simulink model "blade_liebherr_2021_05_26"  (R2020a)
settings: Solver=ode23tb  StartTime=0.0  StopTime=simulation_length  MaxStep=tsample
values from neighbouring files (symbols this model uses):
  tsample = 1e-3    (= 0.001)    [init_liebherr_blade.m]
libraries: nesl_utility x52, fl_lib x31, bichamber_piston_lib x5, fourway_threeland_valve_lib x3, fourway_fourland_valve_lib x2, engine_speed_ctrl_lib x1, Liebherr_Engine_D934_lib x1, pressure_controlled_pump_lib x1
settings Model: SimulationMode=accelerator  Creator=dbagn  LastModifiedBy=dbagn
settings SolverCC: ZeroCrossControl=DisableAll  ZeroCrossAlgorithm=Adaptive
settings DataIOCC: SaveTime=off  ReturnWorkspaceOutputs=off
settings DebuggingCC: IgnoredZcDiagnostic=none
settings SFSimCC: SimParseCustomCode=off

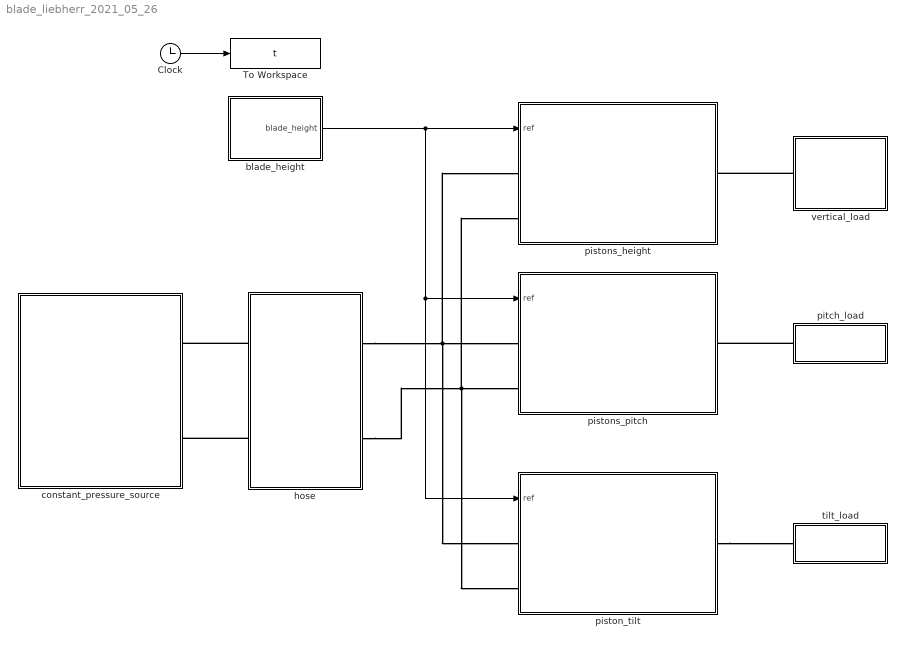
== system blade_liebherr_2021_05_26 ==
  Clock : Clock
  To Workspace : ToWorkspace  VariableName=t  SampleTime=tsample
      settings: MaxDataPoints=Nsample
  blade_height : Subsystem
  constant_pressure_source : Subsystem
  hose : Subsystem
  piston_tilt : Subsystem
  pistons_height : Subsystem
  pistons_pitch : Subsystem
  pitch_load : Subsystem
  tilt_load : Subsystem
  vertical_load : Subsystem
  wires:
  Clock/1 -> To Workspace/1
  blade_height/1(blade_height) -> piston_tilt/1(ref), pistons_pitch/1(ref), pistons_height/1(ref)
  connections:
  hose/LConn1 -- constant_pressure_source/RConn1
  hose/LConn2 -- constant_pressure_source/RConn2
  hose/RConn1 -- piston_tilt/LConn1 -- pistons_height/LConn1 -- pistons_pitch/LConn1
  hose/RConn2 -- piston_tilt/LConn2 -- pistons_height/LConn2 -- pistons_pitch/LConn2
  vertical_load/LConn1 -- pistons_height/RConn1
  pitch_load/RConn1 -- pistons_pitch/RConn1
  piston_tilt/RConn1 -- tilt_load/RConn1

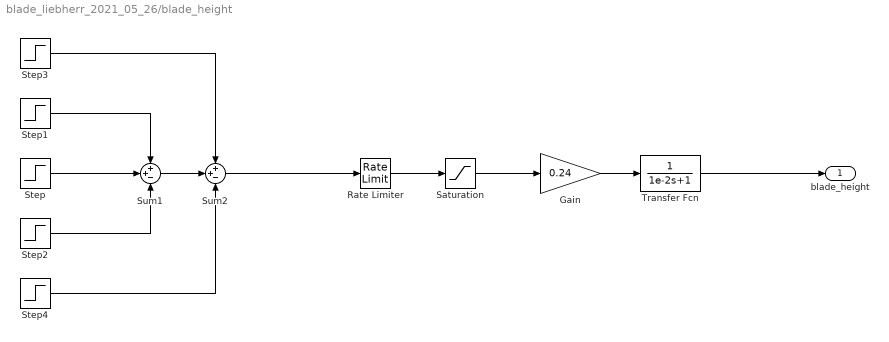
== system blade_liebherr_2021_05_26/blade_height ==
  Gain : Gain  Gain=0.24
  Rate Limiter : RateLimiter  RisingSlewLimit=0.2  FallingSlewLimit=-0.2  SampleTimeMode=inherited
  Saturation : Saturate  UpperLimit=0.99  LowerLimit=-0.99
  Step : Step  Time=20  After=0.5  SampleTime=0
  Step1 : Step  Time=40  SampleTime=0
  Step2 : Step  Time=60  After=2.5  SampleTime=0
  Step3 : Step  Time=80  After=1.4  SampleTime=0
  Step4 : Step  Time=100  After=-0.5  SampleTime=0
  Sum1 : Sum  Inputs=++-
  Sum2 : Sum  Inputs=++-
  Transfer Fcn : TransferFcn  Denominator=[1e-2 1]
  blade_height : Outport
  wires:
  Step/1 -> Sum1/2
  Gain/1 -> Transfer Fcn/1
  Transfer Fcn/1 -> blade_height/1
  Step1/1 -> Sum1/1
  Step2/1 -> Sum1/3
  Sum1/1 -> Sum2/2
  Step3/1 -> Sum2/1
  Step4/1 -> Sum2/3
  Saturation/1 -> Gain/1
  Sum2/1 -> Rate Limiter/1
  Rate Limiter/1 -> Saturation/1

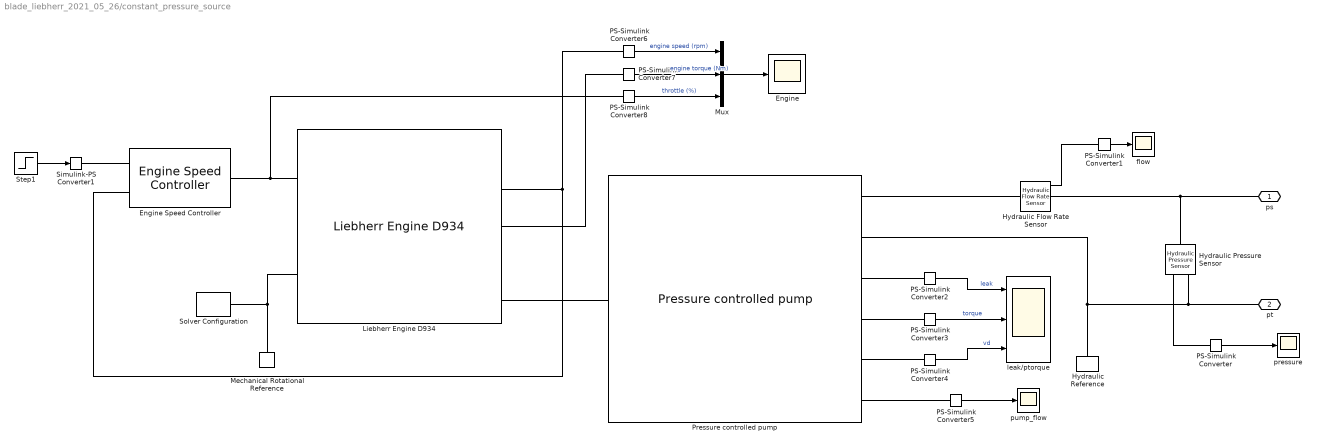
== system blade_liebherr_2021_05_26/constant_pressure_source ==
  Engine : Scope
  Engine Speed Controller : engine_speed_ctrl_lib/Engine Speed Controller  kp=1e-1 s  kint=1e-2  kd=0 s^2  t_out_specify=off  t_out_priority=High  t_out=0  t_out_nominal_specify=off  t_out_nominal_unit=1  t_out_nominal_value=1
      settings: InternalSimscapePortConfiguration="{\"Bottom\":[],\"Left\":[{\"id\":\"we_ref\",\"label\":\"we_ref\",\"type\":\"input\"},{\"id\":\"we\",\"label\":\"we\",\"type\":\"input\"}],\"Right\":[{\"id\":\"theta\",\"label\":\"theta\",\"type\":\"output\"}],\"Top\":[]}"
  Hydraulic Flow Rate Sensor : fl_lib/Hydraulic/Hydraulic Sensors/Hydraulic Flow Rate Sensor
  Hydraulic Pressure Sensor : fl_lib/Hydraulic/Hydraulic Sensors/Hydraulic Pressure Sensor
  Hydraulic Reference : fl_lib/Hydraulic/Hydraulic Elements/Hydraulic Reference
  Liebherr Engine D934 : Liebherr_Engine_D934_lib/Liebherr Engine D934  dynamic_response=simscape.enum.onoff.on  cshaft_inertia=7.5 kg*m^2  initial_speed=600
      settings: InternalSimscapePortConfiguration="{\"Bottom\":[],\"Left\":[{\"id\":\"tS\",\"label\":\"tS\",\"type\":\"input\"},{\"id\":\"C\",\"label\":\"C\",\"type\":\"foundation.mechanical.rotational.rotational\"}],\"Right\":[{\"id\":\"PE\",\"label\":\"PE\",\"type\":\"output\"},{\"id\":\"wE\",\"label\":\"wE\",\"type\":\"output\"},{\"id\":\"tE\",\"label\":\"tE\",\"type\":\"output\"},{\"id\":\"eE\",\"label\":\"eE\",\"type\":\"output\"},{\"id\":\"D\",\"label\":\"D\",\"type\":\"foundation.mechanical.rotational.rotational\"}],\"Top\":[]}"
  Mechanical Rotational Reference : fl_lib/Mechanical/Rotational Elements/Mechanical Rotational Reference
  Mux : Mux  Inputs=3
  PS-Simulink Converter : nesl_utility/PS-Simulink Converter  PhysicalDomain=network_engine_domain  SubClassName=ps_output  LeftPortType=input  RightPortType=output  PseudoPeriodic=off  Frequencies=[]  Unit=bar  AffineConversion=on
  PS-Simulink Converter1 : nesl_utility/PS-Simulink Converter  PhysicalDomain=network_engine_domain  SubClassName=ps_output  LeftPortType=input  RightPortType=output  PseudoPeriodic=off  Frequencies=[]  Unit=l/min  AffineConversion=on
  PS-Simulink Converter{2..5} (4 alike) : nesl_utility/PS-Simulink Converter  PhysicalDomain=network_engine_domain  SubClassName=ps_output  LeftPortType=input  RightPortType=output  PseudoPeriodic=off  Frequencies=[]  Unit=1  AffineConversion=off
  PS-Simulink Converter6 : nesl_utility/PS-Simulink Converter  PhysicalDomain=network_engine_domain  SubClassName=ps_output  LeftPortType=input  RightPortType=output  PseudoPeriodic=off  Frequencies=[]  Unit=inherit  AffineConversion=off
  PS-Simulink Converter7 : nesl_utility/PS-Simulink Converter  PhysicalDomain=network_engine_domain  SubClassName=ps_output  LeftPortType=input  RightPortType=output  PseudoPeriodic=off  Frequencies=[]  Unit=inherit  AffineConversion=off
  PS-Simulink Converter8 : nesl_utility/PS-Simulink Converter  PhysicalDomain=network_engine_domain  SubClassName=ps_output  LeftPortType=input  RightPortType=output  PseudoPeriodic=off  Frequencies=[]  Unit=inherit  AffineConversion=off
  Pressure controlled pump : pressure_controlled_pump_lib/Pressure controlled pump  Vd_nom=62.3*10 cm^3/rev  dp_ref=250 bar  pnom=250 bar  b=0.1 N*m/(rad/s)  inertia_pump=0.027 kg*m^2  vd_lim_max=0.98  vd_lim_min=0  p_set=258 bar  p_reg=8 bar  x_rv_max=12 mm  kpc=8  kic=8 1/s  te_specify=off  te_priority=None  te=0 N*m  te_nominal_specify=off  te_nominal_unit=N*m  te_nominal_value=1  qA_specify=off  qA_priority=None  qA=0 m^3/s  qA_nominal_specify=off  qA_nominal_unit=m^3/s  qA_nominal_value=1  qB_specify=off  qB_priority=None  qB=0 m^3/s  qB_nominal_specify=off  qB_nominal_unit=m^3/s  qB_nominal_value=1  qd_specify=off  qd_priority=None  qd=0 m^3/s  qd_nominal_specify=off  qd_nominal_unit=m^3/s  qd_nominal_value=1  dp_specify=off  dp_priority=None  dp=0 Pa  dp_nominal_specify=off  dp_nominal_unit=Pa  dp_nominal_value=1  vd_specify=off  vd_priority=None  vd=0  vd_nominal_specify=off  vd_nominal_unit=1  vd_nominal_value=1  vd_i_specify=off  vd_i_priority=None  vd_i=0  vd_i_nominal_specify=off  vd_i_nominal_unit=1  vd_i_nominal_value=1  we_specify=off  we_priority=None  we=0 rad/s  we_nominal_specify=off  we_nominal_unit=rad/s  we_nominal_value=1
      settings: InternalSimscapePortConfiguration="{\"Bottom\":[],\"Left\":[{\"id\":\"cW\",\"label\":\"cW\",\"type\":\"foundation.mechanical.rotational.rotational\"}],\"Right\":[{\"id\":\"cA\",\"label\":\"cA\",\"type\":\"foundation.hydraulic.hydraulic\"},{\"id\":\"cB\",\"label\":\"cB\",\"type\":\"foundation.hydraulic.hydraulic\"},{\"id\":\"qleak\",\"label\":\"qleak\",\"type\":\"output\"},{\"id\":\"taup\",\"label\":\"taup\",\"type\":\"output\"},{\"id\":\"vdi\",\"label\":\"vdi\",\"type\":\"output\"},{\"id\":\"pflow\",\"label\":\"pflow\",\"type\":\"output\"}],\"Top\":[]}"
  Simulink-PS Converter1 : nesl_utility/Simulink-PS Converter  PhysicalDomain=network_engine_domain  SubClassName=ps_input  LeftPortType=input  RightPortType=output  PseudoPeriodic=off  Frequencies=[]  NoiseDistribution=none  NoiseParameters=[]  Unit=rpm  AffineConversion=off  FilteringAndDerivatives=zero  SimscapeFilterOrder=2  InputFilterTimeConstant=0.1  UdotUserProvided=0
  Solver Configuration : nesl_utility/Solver Configuration  PhysicalDomain=network_engine_domain  SubClassName=solver  LeftPortType=input  RightPortType=generic  Tones=[]  Harmonics=[]  SimulateNoise=off  Profile=off  UseLocalSampling=off  EnableSwitchedLinearOptims=on  FrequencyDomain=off  UseCCode=off  RelTol=0.001  AbsTol=1e-06  MinStep=1e-09  ToWorkspace=off  RevertToSquareIcSolve=off  NumHomotopyIterations=100  PhasorMode=off  PhasorModeNumHarmonics=1  DoDC=off  ResidualTolerance=1e-09  UseLocalSolver=on  LocalSolverChoice=NE_BACKWARD_EULER_ADVANCER  LocalSolverSampleTime=tsample  DoFixedCost=on  MaxNonlinIter=3  MaxModeIter=2  LinearAlgebra=auto  EquationFormulation=NE_TIME_EF  DelaysMemoryBudget=1024  AutomaticFiltering=on  FilteringTimeConstant=tsample  PartitionStorageMethod=AS_NEEDED  PartitionMemoryBudget=1024  PartitionMethod=ROBUST
  Step1 : Step  Time=0  After=1900  SampleTime=0
  flow : Scope
  leak/ptorque : Scope  NumInputPorts=3
  pressure : Scope
  pump_flow : Scope
  ps : PMIOPort  Side=Right
  pt : PMIOPort  Port=2  Side=Right
  wires:
  PS-Simulink Converter2/1 -> leak/ptorque/1  "leak"
  PS-Simulink Converter/1 -> pressure/1
  PS-Simulink Converter5/1 -> pump_flow/1
  PS-Simulink Converter1/1 -> flow/1
  PS-Simulink Converter3/1 -> leak/ptorque/2  "torque"
  PS-Simulink Converter4/1 -> leak/ptorque/3  "vd"
  Step1/1 -> Simulink-PS Converter1/1
  PS-Simulink Converter6/1 -> Mux/1  "engine speed (rpm)"
  PS-Simulink Converter7/1 -> Mux/2  "engine torque (Nm)"
  Mux/1 -> Engine/1
  PS-Simulink Converter8/1 -> Mux/3  "throttle (%)"
  connections:
  PS-Simulink Converter/LConn1 -- Hydraulic Pressure Sensor/RConn2
  Hydraulic Flow Rate Sensor/RConn2 -- ps/RConn1 -- Hydraulic Pressure Sensor/LConn1
  Pressure controlled pump/RConn6 -- PS-Simulink Converter5/LConn1
  Pressure controlled pump/RConn5 -- PS-Simulink Converter4/LConn1
  Pressure controlled pump/RConn4 -- PS-Simulink Converter3/LConn1
  Hydraulic Flow Rate Sensor/RConn1 -- PS-Simulink Converter1/LConn1
  Pressure controlled pump/RConn1 -- Hydraulic Flow Rate Sensor/LConn1
  Pressure controlled pump/RConn3 -- PS-Simulink Converter2/LConn1
  Pressure controlled pump/LConn1 -- Liebherr Engine D934/RConn5
  Engine Speed Controller/LConn2 -- PS-Simulink Converter6/LConn1 -- Liebherr Engine D934/RConn2
  Engine Speed Controller/LConn1 -- Simulink-PS Converter1/RConn1
  Hydraulic Pressure Sensor/RConn1 -- Pressure controlled pump/RConn2 -- Hydraulic Reference/LConn1 -- pt/RConn1
  PS-Simulink Converter8/LConn1 -- Engine Speed Controller/RConn1 -- Liebherr Engine D934/LConn1
  Mechanical Rotational Reference/LConn1 -- Solver Configuration/RConn1 -- Liebherr Engine D934/LConn2
  PS-Simulink Converter7/LConn1 -- Liebherr Engine D934/RConn3

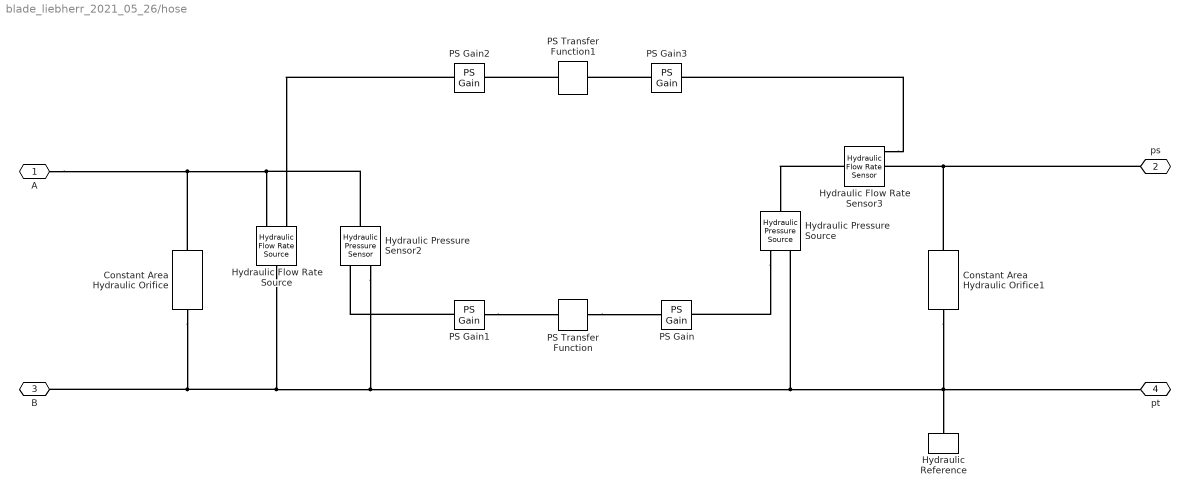
== system blade_liebherr_2021_05_26/hose ==
  Constant Area Hydraulic Orifice : fl_lib/Hydraulic/Hydraulic Elements/Constant Area Hydraulic Orifice  area=1e-8 m^2  C_d=0.7  lam_spec=1  B_lam=0.999  Re_cr=12  q_specify=off  q_priority=None  q=0.001 m^3/s  q_nominal_specify=off  q_nominal_unit=m^3/s  q_nominal_value=1  p_specify=off  p_priority=None  p=0 Pa  p_nominal_specify=off  p_nominal_unit=Pa  p_nominal_value=1
      settings: SourceProductBaseCode=SS  InternalSimscapePortConfiguration="{\"Bottom\":[],\"Left\":[{\"id\":\"A\",\"label\":\"A\",\"type\":\"foundation.hydraulic.hydraulic\"}],\"Right\":[{\"id\":\"B\",\"label\":\"B\",\"type\":\"foundation.hydraulic.hydraulic\"}],\"Top\":[]}"
  Constant Area Hydraulic Orifice1 : fl_lib/Hydraulic/Hydraulic Elements/Constant Area Hydraulic Orifice  area=1e-8 m^2  C_d=0.7  lam_spec=1  B_lam=0.999  Re_cr=12  q_specify=off  q_priority=None  q=0.001 m^3/s  q_nominal_specify=off  q_nominal_unit=m^3/s  q_nominal_value=1  p_specify=off  p_priority=None  p=0 Pa  p_nominal_specify=off  p_nominal_unit=Pa  p_nominal_value=1
      settings: SourceProductBaseCode=SS  InternalSimscapePortConfiguration="{\"Bottom\":[],\"Left\":[{\"id\":\"A\",\"label\":\"A\",\"type\":\"foundation.hydraulic.hydraulic\"}],\"Right\":[{\"id\":\"B\",\"label\":\"B\",\"type\":\"foundation.hydraulic.hydraulic\"}],\"Top\":[]}"
  Hydraulic Flow Rate Sensor3 : fl_lib/Hydraulic/Hydraulic Sensors/Hydraulic Flow Rate Sensor
  Hydraulic Flow Rate Source : fl_lib/Hydraulic/Hydraulic Sources/Hydraulic Flow Rate Source
      settings: SourceProductBaseCode=SS  InternalSimscapePortConfiguration="{\"Bottom\":[],\"Left\":[{\"id\":\"P\",\"label\":\"P\",\"type\":\"foundation.hydraulic.hydraulic\"}],\"Right\":[{\"id\":\"S\",\"label\":\"S\",\"type\":\"input\"},{\"id\":\"T\",\"label\":\"T\",\"type\":\"foundation.hydraulic.hydraulic\"}],\"Top\":[]}"
  Hydraulic Pressure Sensor2 : fl_lib/Hydraulic/Hydraulic Sensors/Hydraulic Pressure Sensor
  Hydraulic Pressure Source : fl_lib/Hydraulic/Hydraulic Sources/Hydraulic Pressure Source
      settings: SourceProductBaseCode=SS  InternalSimscapePortConfiguration="{\"Bottom\":[],\"Left\":[{\"id\":\"P\",\"label\":\"P\",\"type\":\"foundation.hydraulic.hydraulic\"}],\"Right\":[{\"id\":\"S\",\"label\":\"S\",\"type\":\"input\"},{\"id\":\"T\",\"label\":\"T\",\"type\":\"foundation.hydraulic.hydraulic\"}],\"Top\":[]}"
  Hydraulic Reference : fl_lib/Hydraulic/Hydraulic Elements/Hydraulic Reference
  PS Gain : fl_lib/Physical Signals/Functions/PS Gain  gain=1 Pa
  PS Gain1 : fl_lib/Physical Signals/Functions/PS Gain  gain=1 Pa^-1
  PS Gain2 : fl_lib/Physical Signals/Functions/PS Gain  gain=1 m^3/s
  PS Gain3 : fl_lib/Physical Signals/Functions/PS Gain  gain=1 m^-3*s
  PS Transfer Function : fl_lib/Physical Signals/Linear Operators/PS Transfer Function  transfer_function_type=foundation.enum.transfer_function_type.lag  T=0.1 s  T1=2 s  T2=1 s  y0=0
      settings: SourceProductBaseCode=SS  InternalSimscapePortConfiguration="{\"Bottom\":[],\"Left\":[{\"id\":\"U\",\"label\":\"\",\"type\":\"input\"}],\"Right\":[{\"id\":\"Y\",\"label\":\"\",\"type\":\"output\"}],\"Top\":[]}"
  PS Transfer Function1 : fl_lib/Physical Signals/Linear Operators/PS Transfer Function  transfer_function_type=foundation.enum.transfer_function_type.lag  T=0.1 s  T1=2 s  T2=1 s  y0=0
      settings: SourceProductBaseCode=SS  InternalSimscapePortConfiguration="{\"Bottom\":[],\"Left\":[{\"id\":\"U\",\"label\":\"\",\"type\":\"input\"}],\"Right\":[{\"id\":\"Y\",\"label\":\"\",\"type\":\"output\"}],\"Top\":[]}"
  A : PMIOPort  Side=Left
  ps : PMIOPort  Port=2  Side=Right
  B : PMIOPort  Port=3  Side=Left
  pt : PMIOPort  Port=4  Side=Right
  connections:
  ps/RConn1 -- Constant Area Hydraulic Orifice1/LConn1 -- Hydraulic Flow Rate Sensor3/RConn2
  PS Gain2/RConn1 -- Hydraulic Flow Rate Source/RConn1
  Hydraulic Flow Rate Sensor3/RConn1 -- PS Gain3/LConn1
  Hydraulic Flow Rate Sensor3/LConn1 -- Hydraulic Pressure Source/LConn1
  Hydraulic Pressure Source/RConn1 -- PS Gain/RConn1
  PS Gain1/LConn1 -- Hydraulic Pressure Sensor2/RConn2
  Hydraulic Pressure Source/RConn2 -- Hydraulic Pressure Sensor2/RConn1 -- Constant Area Hydraulic Orifice/RConn1 -- B/RConn1 -- Hydraulic Flow Rate Source/LConn1 -- Constant Area Hydraulic Orifice1/RConn1 -- Hydraulic Reference/LConn1 -- pt/RConn1
  PS Transfer Function1/RConn1 -- PS Gain2/LConn1
  PS Transfer Function/RConn1 -- PS Gain/LConn1
  A/RConn1 -- Constant Area Hydraulic Orifice/LConn1 -- Hydraulic Pressure Sensor2/LConn1 -- Hydraulic Flow Rate Source/RConn2
  PS Gain3/RConn1 -- PS Transfer Function1/LConn1
  PS Gain1/RConn1 -- PS Transfer Function/LConn1

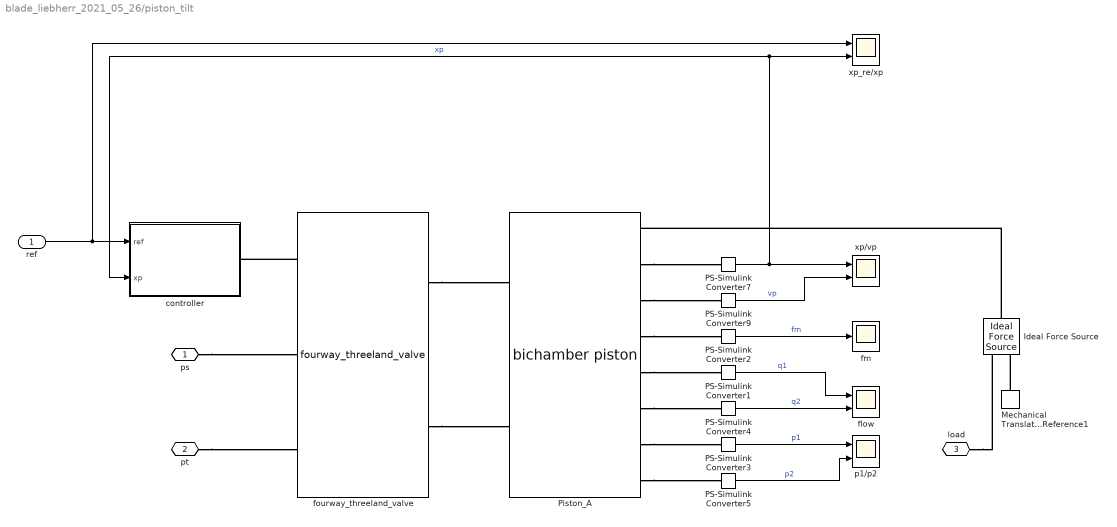
== system blade_liebherr_2021_05_26/piston_tilt ==
  ref : Inport
  Ideal Force Source : fl_lib/Mechanical/Mechanical Sources/Ideal Force Source
  Mechanical Translational Reference1 : fl_lib/Mechanical/Translational Elements/Mechanical Translational Reference
  PS-Simulink Converter{1..5,7,9} (7 alike) : nesl_utility/PS-Simulink Converter  PhysicalDomain=network_engine_domain  SubClassName=ps_output  LeftPortType=input  RightPortType=output  PseudoPeriodic=off  Frequencies=[]  Unit=inherit  AffineConversion=off
  Piston_A : bichamber_piston_lib/bichamber piston  D1=0.08 m  D2=0.08 m  Lp=0.25 m  mp=25 kg  kp=0 N/m  bp=200 N/(m/s)  q1_specify=off  q1_priority=None  q1=0 m^3/s  q1_nominal_specify=off  q1_nominal_unit=m^3/s  q1_nominal_value=1  q2_specify=off  q2_priority=None  q2=0 m^3/s  q2_nominal_specify=off  q2_nominal_unit=m^3/s  q2_nominal_value=1  p1_specify=off  p1_priority=High  p1=0 bar  p1_nominal_specify=off  p1_nominal_unit=bar  p1_nominal_value=1  p2_specify=off  p2_priority=High  p2=0 bar  p2_nominal_specify=off  p2_nominal_unit=bar  p2_nominal_value=1  fp_specify=off  fp_priority=None  fp=0 N  fp_nominal_specify=off  fp_nominal_unit=N  fp_nominal_value=1  vp_specify=off  vp_priority=None  vp=0 m/s  vp_nominal_specify=off  vp_nominal_unit=m/s  vp_nominal_value=1  xp_specify=off  xp_priority=High  xp=0 m  xp_nominal_specify=off  xp_nominal_unit=m  xp_nominal_value=1
      settings: InternalSimscapePortConfiguration="{\"Bottom\":[],\"Left\":[{\"id\":\"H1\",\"label\":\"H1\",\"type\":\"foundation.hydraulic.hydraulic\"},{\"id\":\"H2\",\"label\":\"H2\",\"type\":\"foundation.hydraulic.hydraulic\"}],\"Right\":[{\"id\":\"P\",\"label\":\"P\",\"type\":\"foundation.mechanical.translational.translational\"},{\"id\":\"xp_out\",\"label\":\"xp\",\"type\":\"output\"},{\"id\":\"vp_out\",\"label\":\"vp\",\"type\":\"output\"},{\"id\":\"mforce\",\"label\":\"fm\",\"type\":\"output\"},{\"id\":\"q1_out\",\"label\":\"q1\",\"type\":\"output\"},{\"id\":\"q2_out\",\"label\":\"q2\",\"type\":\"output\"},{\"id\":\"p1_out\",\"label\":\"p1\",\"type\":\"output\"},{\"id\":\"p2_out\",\"label\":\"p2\",\"type\":\"output\"}],\"Top\":[]}"
  controller : Subsystem
  flow : Scope  NumInputPorts=2
  fm : Scope
  fourway_threeland_valve : fourway_threeland_valve_lib/fourway_threeland_valve  xv_max=2.75 mm  q1_specify=off  q1_priority=None  q1=0 m^3/s  q1_nominal_specify=off  q1_nominal_unit=m^3/s  q1_nominal_value=1  q2_specify=off  q2_priority=None  q2=0 m^3/s  q2_nominal_specify=off  q2_nominal_unit=m^3/s  q2_nominal_value=1  qin_specify=off  qin_priority=None  qin=0 m^3/s  qin_nominal_specify=off  qin_nominal_unit=m^3/s  qin_nominal_value=1  qout_specify=off  qout_priority=None  qout=0 m^3/s  qout_nominal_specify=off  qout_nominal_unit=m^3/s  qout_nominal_value=1  p1_specify=off  p1_priority=None  p1=0 bar  p1_nominal_specify=off  p1_nominal_unit=bar  p1_nominal_value=1  p2_specify=off  p2_priority=None  p2=0 bar  p2_nominal_specify=off  p2_nominal_unit=bar  p2_nominal_value=1  ps_specify=off  ps_priority=None  ps=0 bar  ps_nominal_specify=off  ps_nominal_unit=bar  ps_nominal_value=1  pt_specify=off  pt_priority=None  pt=0 bar  pt_nominal_specify=off  pt_nominal_unit=bar  pt_nominal_value=1
      settings: InternalSimscapePortConfiguration="{\"Bottom\":[],\"Left\":[{\"id\":\"xv\",\"label\":\"xv\",\"type\":\"input\"},{\"id\":\"S\",\"label\":\"S\",\"type\":\"foundation.hydraulic.hydraulic\"},{\"id\":\"T\",\"label\":\"T\",\"type\":\"foundation.hydraulic.hydraulic\"}],\"Right\":[{\"id\":\"H1\",\"label\":\"H1\",\"type\":\"foundation.hydraulic.hydraulic\"},{\"id\":\"H2\",\"label\":\"H2\",\"type\":\"foundation.hydraulic.hydraulic\"}],\"Top\":[]}"
  p1/p2 : Scope  NumInputPorts=2
  xp/vp : Scope  NumInputPorts=2
  xp_re/xp : Scope  NumInputPorts=2
  ps : PMIOPort  Side=Left
  pt : PMIOPort  Port=2  Side=Left
  load : PMIOPort  Port=3  Side=Right
  wires:
  ref/1 -> xp_re/xp/1, controller/1(ref)
  PS-Simulink Converter3/1 -> p1/p2/1  "p1"
  PS-Simulink Converter7/1 -> xp_re/xp/2, controller/2(xp), xp/vp/1  "xp"
  PS-Simulink Converter4/1 -> flow/2  "q2"
  PS-Simulink Converter9/1 -> xp/vp/2  "vp"
  PS-Simulink Converter5/1 -> p1/p2/2  "p2"
  PS-Simulink Converter1/1 -> flow/1  "q1"
  PS-Simulink Converter2/1 -> fm/1  "fm"
  connections:
  Mechanical Translational Reference1/LConn1 -- Ideal Force Source/RConn2
  load/RConn1 -- Ideal Force Source/RConn1
  Ideal Force Source/LConn1 -- Piston_A/RConn1
  Piston_A/RConn3 -- PS-Simulink Converter9/LConn1
  fourway_threeland_valve/RConn2 -- Piston_A/LConn2
  fourway_threeland_valve/RConn1 -- Piston_A/LConn1
  Piston_A/RConn2 -- PS-Simulink Converter7/LConn1
  Piston_A/RConn4 -- PS-Simulink Converter2/LConn1
  Piston_A/RConn5 -- PS-Simulink Converter1/LConn1
  Piston_A/RConn6 -- PS-Simulink Converter4/LConn1
  Piston_A/RConn7 -- PS-Simulink Converter3/LConn1
  Piston_A/RConn8 -- PS-Simulink Converter5/LConn1
  ps/RConn1 -- fourway_threeland_valve/LConn2
  pt/RConn1 -- fourway_threeland_valve/LConn3
  fourway_threeland_valve/LConn1 -- controller/RConn1

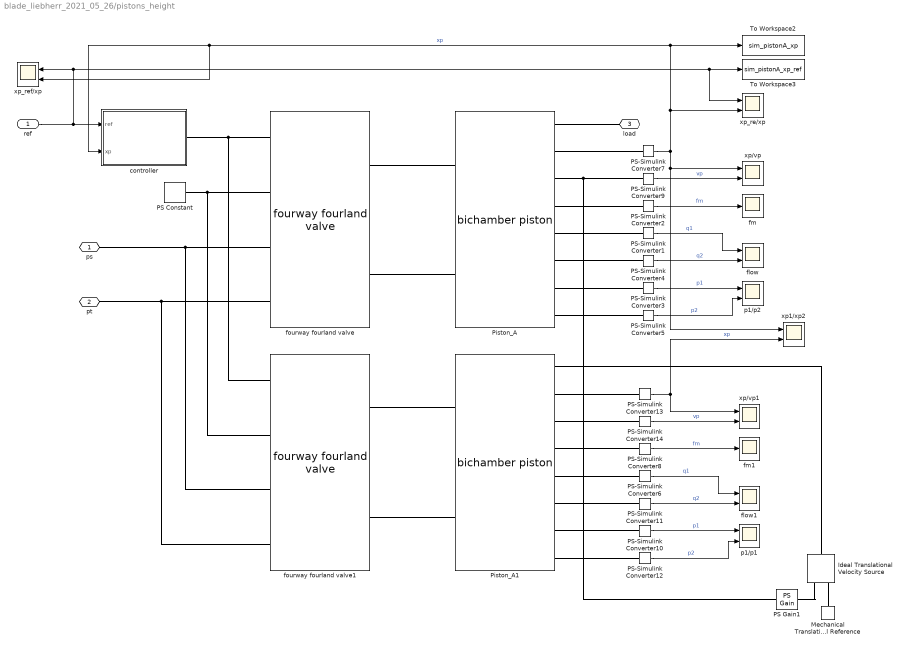
== system blade_liebherr_2021_05_26/pistons_height ==
  ref : Inport
  Ideal Translational Velocity Source : fl_lib/Mechanical/Mechanical Sources/Ideal Translational Velocity Source
  Mechanical Translational Reference : fl_lib/Mechanical/Translational Elements/Mechanical Translational Reference
  PS Constant : fl_lib/Physical Signals/Sources/PS Constant  constant=0 mm
  PS Gain1 : fl_lib/Physical Signals/Functions/PS Gain  gain=1
  PS-Simulink Converter{1..14} (14 alike) : nesl_utility/PS-Simulink Converter  PhysicalDomain=network_engine_domain  SubClassName=ps_output  LeftPortType=input  RightPortType=output  PseudoPeriodic=off  Frequencies=[]  Unit=inherit  AffineConversion=off
  Piston_A : bichamber_piston_lib/bichamber piston  D1=0.08 m  D2=0.08 m  Lp=0.25 m  mp=25 kg  kp=0 N/m  bp=200 N/(m/s)  q1_specify=off  q1_priority=None  q1=0 m^3/s  q1_nominal_specify=off  q1_nominal_unit=m^3/s  q1_nominal_value=1  q2_specify=off  q2_priority=None  q2=0 m^3/s  q2_nominal_specify=off  q2_nominal_unit=m^3/s  q2_nominal_value=1  p1_specify=off  p1_priority=High  p1=0 bar  p1_nominal_specify=off  p1_nominal_unit=bar  p1_nominal_value=1  p2_specify=off  p2_priority=High  p2=0 bar  p2_nominal_specify=off  p2_nominal_unit=bar  p2_nominal_value=1  fp_specify=off  fp_priority=None  fp=0 N  fp_nominal_specify=off  fp_nominal_unit=N  fp_nominal_value=1  vp_specify=off  vp_priority=None  vp=0 m/s  vp_nominal_specify=off  vp_nominal_unit=m/s  vp_nominal_value=1  xp_specify=off  xp_priority=High  xp=0 m  xp_nominal_specify=off  xp_nominal_unit=m  xp_nominal_value=1
      settings: InternalSimscapePortConfiguration="{\"Bottom\":[],\"Left\":[{\"id\":\"H1\",\"label\":\"H1\",\"type\":\"foundation.hydraulic.hydraulic\"},{\"id\":\"H2\",\"label\":\"H2\",\"type\":\"foundation.hydraulic.hydraulic\"}],\"Right\":[{\"id\":\"P\",\"label\":\"P\",\"type\":\"foundation.mechanical.translational.translational\"},{\"id\":\"xp_out\",\"label\":\"xp\",\"type\":\"output\"},{\"id\":\"vp_out\",\"label\":\"vp\",\"type\":\"output\"},{\"id\":\"mforce\",\"label\":\"fm\",\"type\":\"output\"},{\"id\":\"q1_out\",\"label\":\"q1\",\"type\":\"output\"},{\"id\":\"q2_out\",\"label\":\"q2\",\"type\":\"output\"},{\"id\":\"p1_out\",\"label\":\"p1\",\"type\":\"output\"},{\"id\":\"p2_out\",\"label\":\"p2\",\"type\":\"output\"}],\"Top\":[]}"
  Piston_A1 : bichamber_piston_lib/bichamber piston  D1=0.08 m  D2=0.08 m  Lp=0.25 m  mp=25 kg  kp=0 N/m  bp=200 N/(m/s)  q1_specify=off  q1_priority=None  q1=0 m^3/s  q1_nominal_specify=off  q1_nominal_unit=m^3/s  q1_nominal_value=1  q2_specify=off  q2_priority=None  q2=0 m^3/s  q2_nominal_specify=off  q2_nominal_unit=m^3/s  q2_nominal_value=1  p1_specify=off  p1_priority=High  p1=125 bar  p1_nominal_specify=off  p1_nominal_unit=bar  p1_nominal_value=1  p2_specify=off  p2_priority=High  p2=125 bar  p2_nominal_specify=off  p2_nominal_unit=bar  p2_nominal_value=1  fp_specify=off  fp_priority=None  fp=0 N  fp_nominal_specify=off  fp_nominal_unit=N  fp_nominal_value=1  vp_specify=off  vp_priority=None  vp=0 m/s  vp_nominal_specify=off  vp_nominal_unit=m/s  vp_nominal_value=1  xp_specify=off  xp_priority=High  xp=0 m  xp_nominal_specify=off  xp_nominal_unit=m  xp_nominal_value=1
      settings: InternalSimscapePortConfiguration="{\"Bottom\":[],\"Left\":[{\"id\":\"H1\",\"label\":\"H1\",\"type\":\"foundation.hydraulic.hydraulic\"},{\"id\":\"H2\",\"label\":\"H2\",\"type\":\"foundation.hydraulic.hydraulic\"}],\"Right\":[{\"id\":\"P\",\"label\":\"P\",\"type\":\"foundation.mechanical.translational.translational\"},{\"id\":\"xp_out\",\"label\":\"xp\",\"type\":\"output\"},{\"id\":\"vp_out\",\"label\":\"vp\",\"type\":\"output\"},{\"id\":\"mforce\",\"label\":\"fm\",\"type\":\"output\"},{\"id\":\"q1_out\",\"label\":\"q1\",\"type\":\"output\"},{\"id\":\"q2_out\",\"label\":\"q2\",\"type\":\"output\"},{\"id\":\"p1_out\",\"label\":\"p1\",\"type\":\"output\"},{\"id\":\"p2_out\",\"label\":\"p2\",\"type\":\"output\"}],\"Top\":[]}"
  To Workspace2 : ToWorkspace  VariableName=sim_pistonA_xp  SampleTime=tsample
      settings: MaxDataPoints=Nsample
  To Workspace3 : ToWorkspace  VariableName=sim_pistonA_xp_ref  SampleTime=tsample
      settings: MaxDataPoints=Nsample
  controller : Subsystem
  flow : Scope  NumInputPorts=2
  flow1 : Scope  NumInputPorts=2
  fm : Scope
  fm1 : Scope
  fourway fourland valve : fourway_fourland_valve_lib/fourway fourland valve  xv_max=2.75 mm  ps_specify=off  ps_priority=None  ps=0 bar  ps_nominal_specify=off  ps_nominal_unit=bar  ps_nominal_value=1  pt_specify=off  pt_priority=None  pt=0 bar  pt_nominal_specify=off  pt_nominal_unit=bar  pt_nominal_value=1  q1_specify=off  q1_priority=None  q1=0 m^3/s  q1_nominal_specify=off  q1_nominal_unit=m^3/s  q1_nominal_value=1  q2_specify=off  q2_priority=None  q2=0 m^3/s  q2_nominal_specify=off  q2_nominal_unit=m^3/s  q2_nominal_value=1  q3_specify=off  q3_priority=None  q3=0 m^3/s  q3_nominal_specify=off  q3_nominal_unit=m^3/s  q3_nominal_value=1  q4_specify=off  q4_priority=None  q4=0 m^3/s  q4_nominal_specify=off  q4_nominal_unit=m^3/s  q4_nominal_value=1  q5_specify=off  q5_priority=None  q5=0 m^3/s  q5_nominal_specify=off  q5_nominal_unit=m^3/s  q5_nominal_value=1  q6_specify=off  q6_priority=None  q6=0 m^3/s  q6_nominal_specify=off  q6_nominal_unit=m^3/s  q6_nominal_value=1  qs_specify=off  qs_priority=None  qs=0 m^3/s  qs_nominal_specify=off  qs_nominal_unit=m^3/s  qs_nominal_value=1  qt_specify=off  qt_priority=None  qt=0 m^3/s  qt_nominal_specify=off  qt_nominal_unit=m^3/s  qt_nominal_value=1  p1_specify=on  p1_priority=High  p1=125 bar  p1_nominal_specify=off  p1_nominal_unit=bar  p1_nominal_value=1  p2_specify=on  p2_priority=High  p2=125 bar  p2_nominal_specify=off  p2_nominal_unit=bar  p2_nominal_value=1
      settings: InternalSimscapePortConfiguration="{\"Bottom\":[],\"Left\":[{\"id\":\"xv\",\"label\":\"xv\",\"type\":\"input\"},{\"id\":\"x0\",\"label\":\"x0\",\"type\":\"input\"},{\"id\":\"S\",\"label\":\"S\",\"type\":\"foundation.hydraulic.hydraulic\"},{\"id\":\"T\",\"label\":\"T\",\"type\":\"foundation.hydraulic.hydraulic\"}],\"Right\":[{\"id\":\"H1\",\"label\":\"H1\",\"type\":\"foundation.hydraulic.hydraulic\"},{\"id\":\"H2\",\"label\":\"H2\",\"type\":\"foundation.hydraulic.hydraulic\"}],\"Top\":[]}"
  fourway fourland valve1 : fourway_fourland_valve_lib/fourway fourland valve  xv_max=2.75 mm  ps_specify=off  ps_priority=None  ps=0 bar  ps_nominal_specify=off  ps_nominal_unit=bar  ps_nominal_value=1  pt_specify=off  pt_priority=None  pt=0 bar  pt_nominal_specify=off  pt_nominal_unit=bar  pt_nominal_value=1  q1_specify=off  q1_priority=None  q1=0 m^3/s  q1_nominal_specify=off  q1_nominal_unit=m^3/s  q1_nominal_value=1  q2_specify=off  q2_priority=None  q2=0 m^3/s  q2_nominal_specify=off  q2_nominal_unit=m^3/s  q2_nominal_value=1  q3_specify=off  q3_priority=None  q3=0 m^3/s  q3_nominal_specify=off  q3_nominal_unit=m^3/s  q3_nominal_value=1  q4_specify=off  q4_priority=None  q4=0 m^3/s  q4_nominal_specify=off  q4_nominal_unit=m^3/s  q4_nominal_value=1  q5_specify=off  q5_priority=None  q5=0 m^3/s  q5_nominal_specify=off  q5_nominal_unit=m^3/s  q5_nominal_value=1  q6_specify=off  q6_priority=None  q6=0 m^3/s  q6_nominal_specify=off  q6_nominal_unit=m^3/s  q6_nominal_value=1  qs_specify=off  qs_priority=None  qs=0 m^3/s  qs_nominal_specify=off  qs_nominal_unit=m^3/s  qs_nominal_value=1  qt_specify=off  qt_priority=None  qt=0 m^3/s  qt_nominal_specify=off  qt_nominal_unit=m^3/s  qt_nominal_value=1  p1_specify=on  p1_priority=High  p1=125 bar  p1_nominal_specify=off  p1_nominal_unit=bar  p1_nominal_value=1  p2_specify=on  p2_priority=High  p2=125 bar  p2_nominal_specify=off  p2_nominal_unit=bar  p2_nominal_value=1
      settings: InternalSimscapePortConfiguration="{\"Bottom\":[],\"Left\":[{\"id\":\"xv\",\"label\":\"xv\",\"type\":\"input\"},{\"id\":\"x0\",\"label\":\"x0\",\"type\":\"input\"},{\"id\":\"S\",\"label\":\"S\",\"type\":\"foundation.hydraulic.hydraulic\"},{\"id\":\"T\",\"label\":\"T\",\"type\":\"foundation.hydraulic.hydraulic\"}],\"Right\":[{\"id\":\"H1\",\"label\":\"H1\",\"type\":\"foundation.hydraulic.hydraulic\"},{\"id\":\"H2\",\"label\":\"H2\",\"type\":\"foundation.hydraulic.hydraulic\"}],\"Top\":[]}"
  p1/p1 : Scope  NumInputPorts=2
  p1/p2 : Scope  NumInputPorts=2
  xp/vp : Scope  NumInputPorts=2
  xp/vp1 : Scope  NumInputPorts=2
  xp1/xp2 : Scope  NumInputPorts=2
  xp_re/xp : Scope  NumInputPorts=2
  xp_ref/xp : Scope  NumInputPorts=2
  ps : PMIOPort  Side=Left
  pt : PMIOPort  Port=2  Side=Left
  load : PMIOPort  Port=3  Side=Right
  wires:
  ref/1 -> xp_ref/xp/1, xp_re/xp/1, To Workspace3/1, controller/1(ref)
  PS-Simulink Converter3/1 -> p1/p2/1  "p1"
  PS-Simulink Converter7/1 -> controller/2(xp), xp_ref/xp/2, To Workspace2/1, xp_re/xp/2, xp1/xp2/1, xp/vp/1  "xp"
  PS-Simulink Converter4/1 -> flow/2  "q2"
  PS-Simulink Converter9/1 -> xp/vp/2  "vp"
  PS-Simulink Converter5/1 -> p1/p2/2  "p2"
  PS-Simulink Converter1/1 -> flow/1  "q1"
  PS-Simulink Converter2/1 -> fm/1  "fm"
  PS-Simulink Converter8/1 -> fm1/1  "fm"
  PS-Simulink Converter6/1 -> flow1/1  "q1"
  PS-Simulink Converter12/1 -> p1/p1/2  "p2"
  PS-Simulink Converter14/1 -> xp/vp1/2  "vp"
  PS-Simulink Converter11/1 -> flow1/2  "q2"
  PS-Simulink Converter13/1 -> xp1/xp2/2, xp/vp1/1  "xp"
  PS-Simulink Converter10/1 -> p1/p1/1  "p1"
  connections:
  Piston_A/RConn2 -- PS-Simulink Converter7/LConn1
  Piston_A/RConn3 -- PS Gain1/LConn1 -- PS-Simulink Converter9/LConn1
  Piston_A/RConn4 -- PS-Simulink Converter2/LConn1
  Piston_A/RConn5 -- PS-Simulink Converter1/LConn1
  Piston_A/RConn6 -- PS-Simulink Converter4/LConn1
  Piston_A/RConn7 -- PS-Simulink Converter3/LConn1
  Piston_A/RConn8 -- PS-Simulink Converter5/LConn1
  fourway fourland valve/RConn1 -- Piston_A/LConn1
  fourway fourland valve/RConn2 -- Piston_A/LConn2
  ps/RConn1 -- fourway fourland valve1/LConn3 -- fourway fourland valve/LConn3
  pt/RConn1 -- fourway fourland valve1/LConn4 -- fourway fourland valve/LConn4
  controller/RConn1 -- fourway fourland valve1/LConn1 -- fourway fourland valve/LConn1
  PS Constant/RConn1 -- fourway fourland valve/LConn2 -- fourway fourland valve1/LConn2
  Piston_A1/RConn7 -- PS-Simulink Converter10/LConn1
  Piston_A1/RConn5 -- PS-Simulink Converter6/LConn1
  Piston_A1/RConn8 -- PS-Simulink Converter12/LConn1
  Piston_A1/RConn4 -- PS-Simulink Converter8/LConn1
  Piston_A1/RConn2 -- PS-Simulink Converter13/LConn1
  Piston_A1/RConn3 -- PS-Simulink Converter14/LConn1
  Piston_A1/RConn6 -- PS-Simulink Converter11/LConn1
  load/RConn1 -- Piston_A/RConn1
  fourway fourland valve1/RConn1 -- Piston_A1/LConn1
  fourway fourland valve1/RConn2 -- Piston_A1/LConn2
  Ideal Translational Velocity Source/LConn1 -- Piston_A1/RConn1
  Mechanical Translational Reference/LConn1 -- Ideal Translational Velocity Source/RConn2
  PS Gain1/RConn1 -- Ideal Translational Velocity Source/RConn1

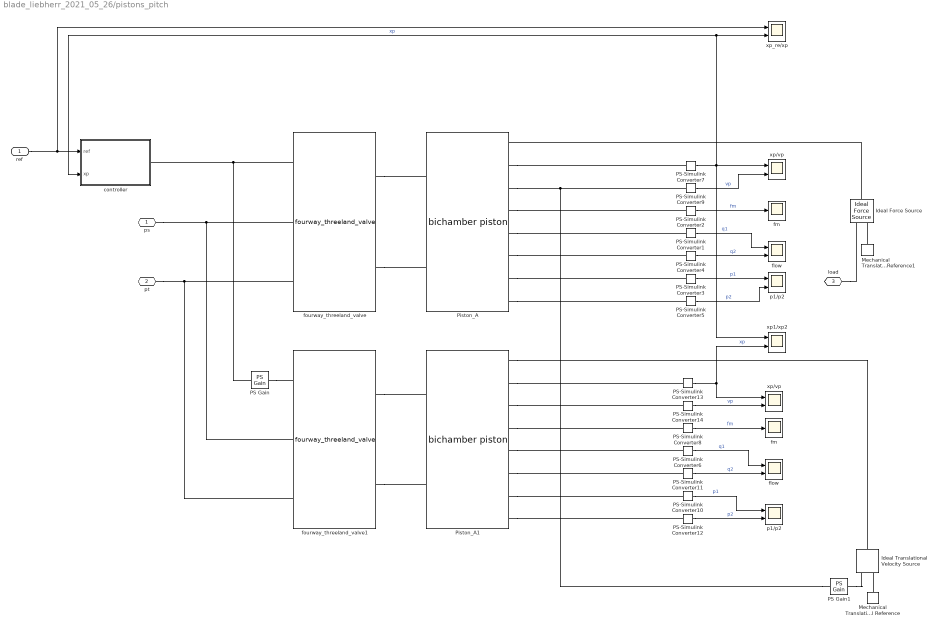
== system blade_liebherr_2021_05_26/pistons_pitch ==
  ref : Inport
  Ideal Force Source : fl_lib/Mechanical/Mechanical Sources/Ideal Force Source
  Ideal Translational Velocity Source : fl_lib/Mechanical/Mechanical Sources/Ideal Translational Velocity Source
  Mechanical Translational Reference : fl_lib/Mechanical/Translational Elements/Mechanical Translational Reference
  Mechanical Translational Reference1 : fl_lib/Mechanical/Translational Elements/Mechanical Translational Reference
  PS Gain : fl_lib/Physical Signals/Functions/PS Gain  gain=-1
  PS Gain1 : fl_lib/Physical Signals/Functions/PS Gain  gain=-1
  PS-Simulink Converter{1..14} (14 alike) : nesl_utility/PS-Simulink Converter  PhysicalDomain=network_engine_domain  SubClassName=ps_output  LeftPortType=input  RightPortType=output  PseudoPeriodic=off  Frequencies=[]  Unit=inherit  AffineConversion=off
  Piston_A : bichamber_piston_lib/bichamber piston  D1=0.08 m  D2=0.08 m  Lp=0.25 m  mp=25 kg  kp=0 N/m  bp=200 N/(m/s)  q1_specify=off  q1_priority=None  q1=0 m^3/s  q1_nominal_specify=off  q1_nominal_unit=m^3/s  q1_nominal_value=1  q2_specify=off  q2_priority=None  q2=0 m^3/s  q2_nominal_specify=off  q2_nominal_unit=m^3/s  q2_nominal_value=1  p1_specify=off  p1_priority=High  p1=0 bar  p1_nominal_specify=off  p1_nominal_unit=bar  p1_nominal_value=1  p2_specify=off  p2_priority=High  p2=0 bar  p2_nominal_specify=off  p2_nominal_unit=bar  p2_nominal_value=1  fp_specify=off  fp_priority=None  fp=0 N  fp_nominal_specify=off  fp_nominal_unit=N  fp_nominal_value=1  vp_specify=off  vp_priority=None  vp=0 m/s  vp_nominal_specify=off  vp_nominal_unit=m/s  vp_nominal_value=1  xp_specify=off  xp_priority=High  xp=0 m  xp_nominal_specify=off  xp_nominal_unit=m  xp_nominal_value=1
      settings: InternalSimscapePortConfiguration="{\"Bottom\":[],\"Left\":[{\"id\":\"H1\",\"label\":\"H1\",\"type\":\"foundation.hydraulic.hydraulic\"},{\"id\":\"H2\",\"label\":\"H2\",\"type\":\"foundation.hydraulic.hydraulic\"}],\"Right\":[{\"id\":\"P\",\"label\":\"P\",\"type\":\"foundation.mechanical.translational.translational\"},{\"id\":\"xp_out\",\"label\":\"xp\",\"type\":\"output\"},{\"id\":\"vp_out\",\"label\":\"vp\",\"type\":\"output\"},{\"id\":\"mforce\",\"label\":\"fm\",\"type\":\"output\"},{\"id\":\"q1_out\",\"label\":\"q1\",\"type\":\"output\"},{\"id\":\"q2_out\",\"label\":\"q2\",\"type\":\"output\"},{\"id\":\"p1_out\",\"label\":\"p1\",\"type\":\"output\"},{\"id\":\"p2_out\",\"label\":\"p2\",\"type\":\"output\"}],\"Top\":[]}"
  Piston_A1 : bichamber_piston_lib/bichamber piston  D1=0.08 m  D2=0.08 m  Lp=0.25 m  mp=25 kg  kp=0 N/m  bp=200 N/(m/s)  q1_specify=off  q1_priority=None  q1=0 m^3/s  q1_nominal_specify=off  q1_nominal_unit=m^3/s  q1_nominal_value=1  q2_specify=off  q2_priority=None  q2=0 m^3/s  q2_nominal_specify=off  q2_nominal_unit=m^3/s  q2_nominal_value=1  p1_specify=off  p1_priority=High  p1=0 bar  p1_nominal_specify=off  p1_nominal_unit=bar  p1_nominal_value=1  p2_specify=off  p2_priority=High  p2=0 bar  p2_nominal_specify=off  p2_nominal_unit=bar  p2_nominal_value=1  fp_specify=off  fp_priority=None  fp=0 N  fp_nominal_specify=off  fp_nominal_unit=N  fp_nominal_value=1  vp_specify=off  vp_priority=None  vp=0 m/s  vp_nominal_specify=off  vp_nominal_unit=m/s  vp_nominal_value=1  xp_specify=off  xp_priority=High  xp=0 m  xp_nominal_specify=off  xp_nominal_unit=m  xp_nominal_value=1
      settings: InternalSimscapePortConfiguration="{\"Bottom\":[],\"Left\":[{\"id\":\"H1\",\"label\":\"H1\",\"type\":\"foundation.hydraulic.hydraulic\"},{\"id\":\"H2\",\"label\":\"H2\",\"type\":\"foundation.hydraulic.hydraulic\"}],\"Right\":[{\"id\":\"P\",\"label\":\"P\",\"type\":\"foundation.mechanical.translational.translational\"},{\"id\":\"xp_out\",\"label\":\"xp\",\"type\":\"output\"},{\"id\":\"vp_out\",\"label\":\"vp\",\"type\":\"output\"},{\"id\":\"mforce\",\"label\":\"fm\",\"type\":\"output\"},{\"id\":\"q1_out\",\"label\":\"q1\",\"type\":\"output\"},{\"id\":\"q2_out\",\"label\":\"q2\",\"type\":\"output\"},{\"id\":\"p1_out\",\"label\":\"p1\",\"type\":\"output\"},{\"id\":\"p2_out\",\"label\":\"p2\",\"type\":\"output\"}],\"Top\":[]}"
  controller : Subsystem
  flow : Scope  NumInputPorts=2
  "flow " : Scope  NumInputPorts=2
  fm : Scope
  "fm " : Scope
  fourway_threeland_valve : fourway_threeland_valve_lib/fourway_threeland_valve  xv_max=2.75 mm  q1_specify=off  q1_priority=None  q1=0 m^3/s  q1_nominal_specify=off  q1_nominal_unit=m^3/s  q1_nominal_value=1  q2_specify=off  q2_priority=None  q2=0 m^3/s  q2_nominal_specify=off  q2_nominal_unit=m^3/s  q2_nominal_value=1  qin_specify=off  qin_priority=None  qin=0 m^3/s  qin_nominal_specify=off  qin_nominal_unit=m^3/s  qin_nominal_value=1  qout_specify=off  qout_priority=None  qout=0 m^3/s  qout_nominal_specify=off  qout_nominal_unit=m^3/s  qout_nominal_value=1  p1_specify=off  p1_priority=None  p1=0 bar  p1_nominal_specify=off  p1_nominal_unit=bar  p1_nominal_value=1  p2_specify=off  p2_priority=None  p2=0 bar  p2_nominal_specify=off  p2_nominal_unit=bar  p2_nominal_value=1  ps_specify=off  ps_priority=None  ps=0 bar  ps_nominal_specify=off  ps_nominal_unit=bar  ps_nominal_value=1  pt_specify=off  pt_priority=None  pt=0 bar  pt_nominal_specify=off  pt_nominal_unit=bar  pt_nominal_value=1
      settings: InternalSimscapePortConfiguration="{\"Bottom\":[],\"Left\":[{\"id\":\"xv\",\"label\":\"xv\",\"type\":\"input\"},{\"id\":\"S\",\"label\":\"S\",\"type\":\"foundation.hydraulic.hydraulic\"},{\"id\":\"T\",\"label\":\"T\",\"type\":\"foundation.hydraulic.hydraulic\"}],\"Right\":[{\"id\":\"H1\",\"label\":\"H1\",\"type\":\"foundation.hydraulic.hydraulic\"},{\"id\":\"H2\",\"label\":\"H2\",\"type\":\"foundation.hydraulic.hydraulic\"}],\"Top\":[]}"
  fourway_threeland_valve1 : fourway_threeland_valve_lib/fourway_threeland_valve  xv_max=2.75 mm  q1_specify=off  q1_priority=None  q1=0 m^3/s  q1_nominal_specify=off  q1_nominal_unit=m^3/s  q1_nominal_value=1  q2_specify=off  q2_priority=None  q2=0 m^3/s  q2_nominal_specify=off  q2_nominal_unit=m^3/s  q2_nominal_value=1  qin_specify=off  qin_priority=None  qin=0 m^3/s  qin_nominal_specify=off  qin_nominal_unit=m^3/s  qin_nominal_value=1  qout_specify=off  qout_priority=None  qout=0 m^3/s  qout_nominal_specify=off  qout_nominal_unit=m^3/s  qout_nominal_value=1  p1_specify=off  p1_priority=None  p1=0 bar  p1_nominal_specify=off  p1_nominal_unit=bar  p1_nominal_value=1  p2_specify=off  p2_priority=None  p2=0 bar  p2_nominal_specify=off  p2_nominal_unit=bar  p2_nominal_value=1  ps_specify=off  ps_priority=None  ps=0 bar  ps_nominal_specify=off  ps_nominal_unit=bar  ps_nominal_value=1  pt_specify=off  pt_priority=None  pt=0 bar  pt_nominal_specify=off  pt_nominal_unit=bar  pt_nominal_value=1
      settings: InternalSimscapePortConfiguration="{\"Bottom\":[],\"Left\":[{\"id\":\"xv\",\"label\":\"xv\",\"type\":\"input\"},{\"id\":\"S\",\"label\":\"S\",\"type\":\"foundation.hydraulic.hydraulic\"},{\"id\":\"T\",\"label\":\"T\",\"type\":\"foundation.hydraulic.hydraulic\"}],\"Right\":[{\"id\":\"H1\",\"label\":\"H1\",\"type\":\"foundation.hydraulic.hydraulic\"},{\"id\":\"H2\",\"label\":\"H2\",\"type\":\"foundation.hydraulic.hydraulic\"}],\"Top\":[]}"
  p1/p2 : Scope  NumInputPorts=2
  "p1/p2 " : Scope  NumInputPorts=2
  xp/vp : Scope  NumInputPorts=2
  "xp/vp " : Scope  NumInputPorts=2
  xp1/xp2 : Scope  NumInputPorts=2
  xp_re/xp : Scope  NumInputPorts=2
  ps : PMIOPort  Side=Left
  pt : PMIOPort  Port=2  Side=Left
  load : PMIOPort  Port=3  Side=Right
  wires:
  PS-Simulink Converter10/1 -> "p1/p2 "/1  "p1"
  PS-Simulink Converter13/1 -> xp1/xp2/2, "xp/vp "/1  "xp"
  PS-Simulink Converter11/1 -> "flow "/2  "q2"
  PS-Simulink Converter14/1 -> "xp/vp "/2  "vp"
  PS-Simulink Converter12/1 -> "p1/p2 "/2  "p2"
  PS-Simulink Converter6/1 -> "flow "/1  "q1"
  PS-Simulink Converter8/1 -> "fm "/1  "fm"
  PS-Simulink Converter2/1 -> fm/1  "fm"
  PS-Simulink Converter1/1 -> flow/1  "q1"
  PS-Simulink Converter5/1 -> p1/p2/2  "p2"
  PS-Simulink Converter9/1 -> xp/vp/2  "vp"
  PS-Simulink Converter4/1 -> flow/2  "q2"
  PS-Simulink Converter7/1 -> xp1/xp2/1, xp/vp/1, controller/2(xp), xp_re/xp/2  "xp"
  PS-Simulink Converter3/1 -> p1/p2/1  "p1"
  ref/1 -> controller/1(ref), xp_re/xp/1
  connections:
  Piston_A1/RConn6 -- PS-Simulink Converter11/LConn1
  Piston_A1/RConn3 -- PS-Simulink Converter14/LConn1
  Piston_A1/RConn2 -- PS-Simulink Converter13/LConn1
  Piston_A1/RConn4 -- PS-Simulink Converter8/LConn1
  Piston_A1/RConn8 -- PS-Simulink Converter12/LConn1
  Piston_A1/RConn5 -- PS-Simulink Converter6/LConn1
  Piston_A1/RConn7 -- PS-Simulink Converter10/LConn1
  fourway_threeland_valve/LConn1 -- PS Gain/LConn1 -- controller/RConn1
  pt/RConn1 -- fourway_threeland_valve/LConn3 -- fourway_threeland_valve1/LConn3
  ps/RConn1 -- fourway_threeland_valve/LConn2 -- fourway_threeland_valve1/LConn2
  Piston_A/RConn8 -- PS-Simulink Converter5/LConn1
  Piston_A/RConn7 -- PS-Simulink Converter3/LConn1
  Piston_A/RConn6 -- PS-Simulink Converter4/LConn1
  Piston_A/RConn5 -- PS-Simulink Converter1/LConn1
  Piston_A/RConn4 -- PS-Simulink Converter2/LConn1
  PS Gain1/RConn1 -- Ideal Translational Velocity Source/RConn1
  Piston_A/RConn2 -- PS-Simulink Converter7/LConn1
  fourway_threeland_valve/RConn1 -- Piston_A/LConn1
  fourway_threeland_valve/RConn2 -- Piston_A/LConn2
  fourway_threeland_valve1/RConn1 -- Piston_A1/LConn1
  fourway_threeland_valve1/RConn2 -- Piston_A1/LConn2
  PS Gain/RConn1 -- fourway_threeland_valve1/LConn1
  PS Gain1/LConn1 -- PS-Simulink Converter9/LConn1 -- Piston_A/RConn3
  Mechanical Translational Reference/LConn1 -- Ideal Translational Velocity Source/RConn2
  Ideal Force Source/LConn1 -- Piston_A/RConn1
  load/RConn1 -- Ideal Force Source/RConn1
  Mechanical Translational Reference1/LConn1 -- Ideal Force Source/RConn2
  Piston_A1/RConn1 -- Ideal Translational Velocity Source/LConn1

== system blade_liebherr_2021_05_26/pitch_load ==
  Simulink-PS Converter1 : nesl_utility/Simulink-PS Converter  PhysicalDomain=network_engine_domain  SubClassName=ps_input  LeftPortType=input  RightPortType=output  PseudoPeriodic=off  Frequencies=[]  NoiseDistribution=none  NoiseParameters=[]  Unit=N  AffineConversion=on  FilteringAndDerivatives=provide  SimscapeFilterOrder=1  InputFilterTimeConstant=0.001  UdotUserProvided=0
  "yaw_load  " : Subsystem
  load : PMIOPort  Side=Right
  wires:
  "yaw_load  "/1(Out1) -> Simulink-PS Converter1/1  "yaw_load"
  connections:
  load/RConn1 -- Simulink-PS Converter1/RConn1

== system blade_liebherr_2021_05_26/tilt_load ==
  Simulink-PS Converter1 : nesl_utility/Simulink-PS Converter  PhysicalDomain=network_engine_domain  SubClassName=ps_input  LeftPortType=input  RightPortType=output  PseudoPeriodic=off  Frequencies=[]  NoiseDistribution=none  NoiseParameters=[]  Unit=N  AffineConversion=on  FilteringAndDerivatives=provide  SimscapeFilterOrder=1  InputFilterTimeConstant=0.001  UdotUserProvided=0
  "yaw_load  " : Subsystem
  load : PMIOPort  Side=Right
  wires:
  "yaw_load  "/1(Out1) -> Simulink-PS Converter1/1  "yaw_load"
  connections:
  load/RConn1 -- Simulink-PS Converter1/RConn1

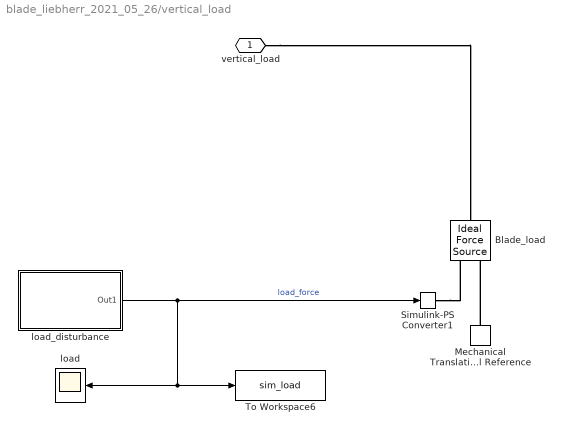
== system blade_liebherr_2021_05_26/vertical_load ==
  Blade_load : fl_lib/Mechanical/Mechanical Sources/Ideal Force Source
  Mechanical Translational Reference : fl_lib/Mechanical/Translational Elements/Mechanical Translational Reference
  Simulink-PS Converter1 : nesl_utility/Simulink-PS Converter  PhysicalDomain=network_engine_domain  SubClassName=ps_input  LeftPortType=input  RightPortType=output  PseudoPeriodic=off  Frequencies=[]  NoiseDistribution=none  NoiseParameters=[]  Unit=N  AffineConversion=on  FilteringAndDerivatives=provide  SimscapeFilterOrder=1  InputFilterTimeConstant=0.001  UdotUserProvided=0
  To Workspace6 : ToWorkspace  VariableName=sim_load  SampleTime=tsample
      settings: MaxDataPoints=Nsample
  load : Scope
  load_disturbance : Subsystem
  vertical_load : PMIOPort  Side=Left
  wires:
  load_disturbance/1(Out1) -> load/1, To Workspace6/1, Simulink-PS Converter1/1  "load_force"
  connections:
  Mechanical Translational Reference/LConn1 -- Blade_load/RConn2
  Simulink-PS Converter1/RConn1 -- Blade_load/RConn1
  vertical_load/RConn1 -- Blade_load/LConn1

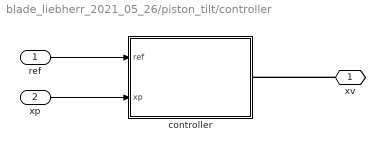
== system blade_liebherr_2021_05_26/piston_tilt/controller ==
  ref : Inport
  xp : Inport  Port=2
  controller : Subsystem
  xv : PMIOPort  Side=Right
  wires:
  ref/1 -> controller/1(ref)
  xp/1 -> controller/2(xp)
  connections:
  xv/RConn1 -- controller/RConn1

== system blade_liebherr_2021_05_26/pistons_height/controller ==
  ref : Inport
  xp : Inport  Port=2
  controller : Subsystem
  xv : PMIOPort  Side=Right
  wires:
  ref/1 -> controller/1(ref)
  xp/1 -> controller/2(xp)
  connections:
  xv/RConn1 -- controller/RConn1

== system blade_liebherr_2021_05_26/pistons_pitch/controller ==
  ref : Inport
  xp : Inport  Port=2
  controller : Subsystem
  xv : PMIOPort  Side=Right
  wires:
  xp/1 -> controller/2(xp)
  ref/1 -> controller/1(ref)
  connections:
  xv/RConn1 -- controller/RConn1

== system blade_liebherr_2021_05_26/pitch_load/yaw_load   ==
  Gain1 : Gain
  Step7 : Step  Time=10  After=15700  SampleTime=0
  Transfer Fcn : TransferFcn  Denominator=[1e-1 1]
  Out1 : Outport
  wires:
  Gain1/1 -> Transfer Fcn/1
  Step7/1 -> Gain1/1
  Transfer Fcn/1 -> Out1/1

== system blade_liebherr_2021_05_26/tilt_load/yaw_load   ==
  Gain1 : Gain
  Step7 : Step  Time=10  After=15700  SampleTime=0
  Transfer Fcn : TransferFcn  Denominator=[1e-1 1]
  Out1 : Outport
  wires:
  Transfer Fcn/1 -> Out1/1
  Step7/1 -> Gain1/1
  Gain1/1 -> Transfer Fcn/1

== system blade_liebherr_2021_05_26/vertical_load/load_disturbance ==
  Gain1 : Gain  Gain=5
  Step7 : Step  Time=10  After=15700  SampleTime=0
  Transfer Fcn : TransferFcn  Denominator=[1e-1 1]
  Out1 : Outport
  wires:
  Gain1/1 -> Transfer Fcn/1
  Step7/1 -> Gain1/1
  Transfer Fcn/1 -> Out1/1

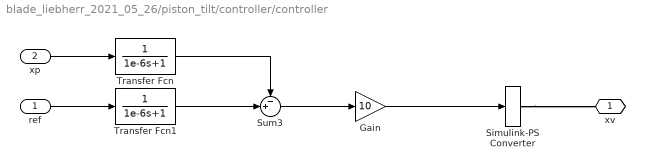
== system blade_liebherr_2021_05_26/piston_tilt/controller/controller ==
  ref : Inport
  xp : Inport  Port=2
  Gain : Gain  Gain=10
  Simulink-PS Converter : nesl_utility/Simulink-PS Converter  PhysicalDomain=network_engine_domain  SubClassName=ps_input  LeftPortType=input  RightPortType=output  PseudoPeriodic=off  Frequencies=[]  NoiseDistribution=none  NoiseParameters=[]  Unit=mm  AffineConversion=on  FilteringAndDerivatives=provide  SimscapeFilterOrder=2  InputFilterTimeConstant=0.025  UdotUserProvided=0
  Sum3 : Sum  Inputs=-+|
  Transfer Fcn : TransferFcn  Denominator=[1e-6 1]
  Transfer Fcn1 : TransferFcn  Denominator=[1e-6 1]
  xv : PMIOPort  Side=Right
  wires:
  Transfer Fcn1/1 -> Sum3/2
  xp/1 -> Transfer Fcn/1
  ref/1 -> Transfer Fcn1/1
  Sum3/1 -> Gain/1
  Transfer Fcn/1 -> Sum3/1
  Gain/1 -> Simulink-PS Converter/1
  connections:
  Simulink-PS Converter/RConn1 -- xv/RConn1

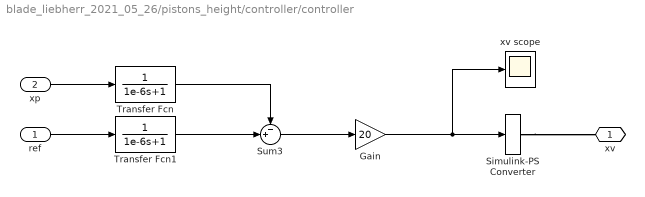
== system blade_liebherr_2021_05_26/pistons_height/controller/controller ==
  ref : Inport
  xp : Inport  Port=2
  Gain : Gain  Gain=20
  Simulink-PS Converter : nesl_utility/Simulink-PS Converter  PhysicalDomain=network_engine_domain  SubClassName=ps_input  LeftPortType=input  RightPortType=output  PseudoPeriodic=off  Frequencies=[]  NoiseDistribution=none  NoiseParameters=[]  Unit=mm  AffineConversion=on  FilteringAndDerivatives=provide  SimscapeFilterOrder=2  InputFilterTimeConstant=0.025  UdotUserProvided=0
  Sum3 : Sum  Inputs=-+|
  Transfer Fcn : TransferFcn  Denominator=[1e-6 1]
  Transfer Fcn1 : TransferFcn  Denominator=[1e-6 1]
  xv scope : Scope
  xv : PMIOPort  Side=Right
  wires:
  xp/1 -> Transfer Fcn/1
  ref/1 -> Transfer Fcn1/1
  Sum3/1 -> Gain/1
  Transfer Fcn/1 -> Sum3/1
  Gain/1 -> xv scope/1, Simulink-PS Converter/1
  Transfer Fcn1/1 -> Sum3/2
  connections:
  Simulink-PS Converter/RConn1 -- xv/RConn1

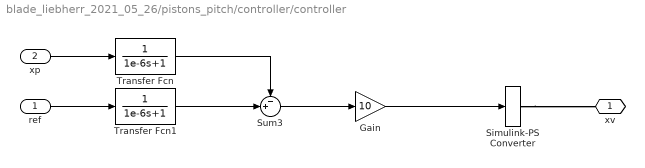
== system blade_liebherr_2021_05_26/pistons_pitch/controller/controller ==
  ref : Inport
  xp : Inport  Port=2
  Gain : Gain  Gain=10
  Simulink-PS Converter : nesl_utility/Simulink-PS Converter  PhysicalDomain=network_engine_domain  SubClassName=ps_input  LeftPortType=input  RightPortType=output  PseudoPeriodic=off  Frequencies=[]  NoiseDistribution=none  NoiseParameters=[]  Unit=mm  AffineConversion=on  FilteringAndDerivatives=provide  SimscapeFilterOrder=2  InputFilterTimeConstant=0.025  UdotUserProvided=0
  Sum3 : Sum  Inputs=-+|
  Transfer Fcn : TransferFcn  Denominator=[1e-6 1]
  Transfer Fcn1 : TransferFcn  Denominator=[1e-6 1]
  xv : PMIOPort  Side=Right
  wires:
  Gain/1 -> Simulink-PS Converter/1
  Transfer Fcn/1 -> Sum3/1
  Sum3/1 -> Gain/1
  ref/1 -> Transfer Fcn1/1
  xp/1 -> Transfer Fcn/1
  Transfer Fcn1/1 -> Sum3/2
  connections:
  Simulink-PS Converter/RConn1 -- xv/RConn1
